simulink model "otimizacao_inercia_final"  (R2023b)
settings: Solver=ode14x  StartTime=0.0  StopTime=10  FixedStep=0.001  RelTol=1e-3  AbsTol=1e-3
values from neighbouring files (symbols this model uses):
  AnguloReal = AnguloR(33:788,1)    [otimizacao_inercia_fmincon.m]    (also in otimizacao_inercia_fminsearch.m)
  c = parametros (2)    [erro_inercia_novo.m]
  g = 9.8    [otimizacao_inercia_fmincon.m]    (also in otimizacao_inercia_fminsearch.m)
  J = parametros (1)    [erro_inercia_novo.m]
  l = 0.38    [otimizacao_inercia_fmincon.m]    (also in otimizacao_inercia_fminsearch.m)
  m = 0.099    [otimizacao_inercia_fmincon.m]    (also in otimizacao_inercia_fminsearch.m)
  TemposR = t(33:788,1)-t(33,1)    [otimizacao_inercia_fmincon.m]    (also in otimizacao_inercia_fminsearch.m)
libraries: simulink_extras x1
settings Model: Creator=henri  LastModifiedBy=alexa
settings SolverCC: AutoScaleAbsTol=off  AlgebraicLoopSolver=TrustRegion  MaxZcPerStep=1
settings DebuggingCC: UnconnectedInputMsg=warning  UnconnectedOutputMsg=warning  UnconnectedLineMsg=warning  SymbolicDimsDataTypeCodeGenerationDiagnostic=none
settings ModelReferenceCC: EnableRefExpFcnMdlSchedulingChecks=on
settings SFSimCC: CustomCodeUndefinedFunction=UseInterfaceOnly
settings RTWCC: DLArmComputeVersion=19.05
settings SimscapeCC: SimscapeLogType=all  SimscapeLogSimulationStatistics=on  SimscapeLogDataHistory=10000

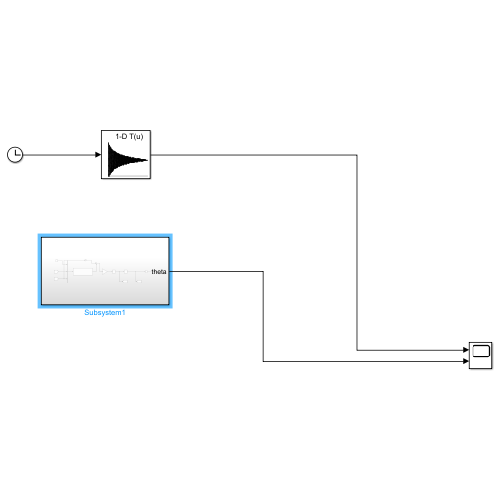
[thumbnail: Simulink's stored preview of the top-level diagram]
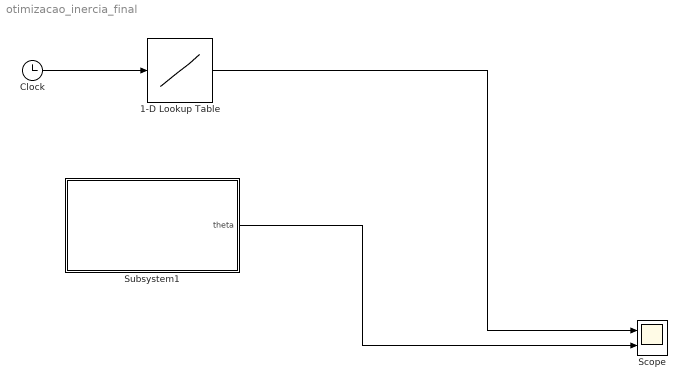
== system otimizacao_inercia_final ==
  1-D Lookup Table : Lookup_n-D  NumberOfTableDimensions=1  BreakpointsForDimension1=TemposR  Table=AnguloReal  InternalRulePriority=Speed  RndMeth=Simplest
  Clock : Clock
  Scope : Scope  NumInputPorts=2
  Subsystem1 : Subsystem
  wires:
  Clock/1 -> 1-D Lookup Table/1
  1-D Lookup Table/1 -> Scope/1
  Subsystem1/1(theta) -> Scope/2

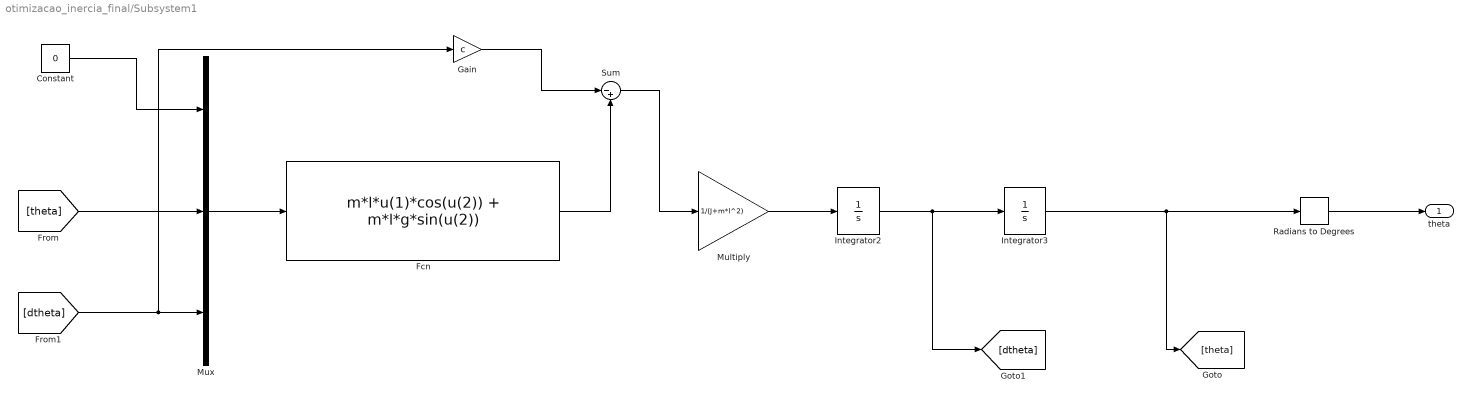
== system otimizacao_inercia_final/Subsystem1 ==
  Constant : Constant  Value=0
  Fcn : Fcn  Expr=m*l*u(1)*cos(u(2)) + m*l*g*sin(u(2))
  Gain : Gain  Gain=c
  Integrator2 : Integrator
  Integrator3 : Integrator  InitialCondition=328*pi/180
  Multiply : Gain  Gain=1/(J+m*l^2)
  Mux : Mux  Inputs=3
  Radians to Degrees : simulink_extras/Transformations/Radians to Degrees
  Sum : Sum  Inputs=|-+
  theta : Outport
  wires:
  Fcn/1 -> Sum/2
  [theta] -> Mux/2
  Mux/1 -> Fcn/1
  [dtheta] -> Gain/1, Mux/3
  Multiply/1 -> Integrator2/1
  Integrator2/1 -> Integrator3/1, [dtheta]
  Integrator3/1 -> Radians to Degrees/1, [theta]
  Radians to Degrees/1 -> theta/1
  Constant/1 -> Mux/1
  Gain/1 -> Sum/1
  Sum/1 -> Multiply/1
